simulink model "simulink_mppt_model"  (R2022b)
settings: Solver=VariableStepAuto  StartTime=0.0  StopTime=60  RelTol=1e-3  AbsTol=1e-3
model workspace (MAT data in the model file):
  Fsw = 40000
  Kc = 832.120994276
  batteryVoltage = 130
  deadTime = 5e-08
  wp = 45312.8685633
  wz = 3484.96300111
  zeroConductanceDef = 0.1
  zeroCurrentDef = 0.05
  zeroVoltageDef = 0.1
undefined symbols (not defined in the file): Ion, Lithium, sigbuilder_block
libraries: spsSeriesRLCBranchLib x5, dspstat3 x3, spsBatteryLib x1, spsControlledCurrentSourceLib x1, spsPVArrayLib x1, spsBoostConverterLib x1, spspowerguiLib x1
settings Model: ParameterArgumentNames=Fsw,deadTime,zeroCurrentDef  Creator=maxim  LastModifiedBy=maxim
settings SolverCC: AutoScaleAbsTol=off  AlgebraicLoopSolver=TrustRegion  MaxZcPerStep=1
settings DebuggingCC: UnconnectedInputMsg=warning  UnconnectedOutputMsg=warning  UnconnectedLineMsg=warning  SymbolicDimsDataTypeCodeGenerationDiagnostic=none  SFMachineParentedDataDiag=warning
settings ModelReferenceCC: EnableRefExpFcnMdlSchedulingChecks=on
settings SFSimCC: CustomCodeUndefinedFunction=UseInterfaceOnly  SimTargetLang=C++
settings RTWCC: DLArmComputeVersion=19.05
settings SimscapeCC: SimscapeLogType=all  SimscapeLogSimulationStatistics=on  SimscapeLogDataHistory=10000

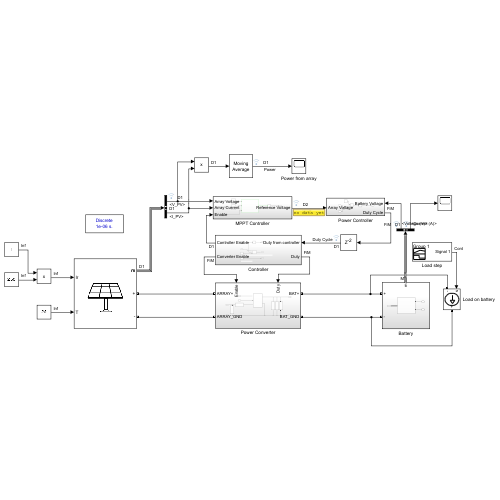
[thumbnail: Simulink's stored preview of the top-level diagram]
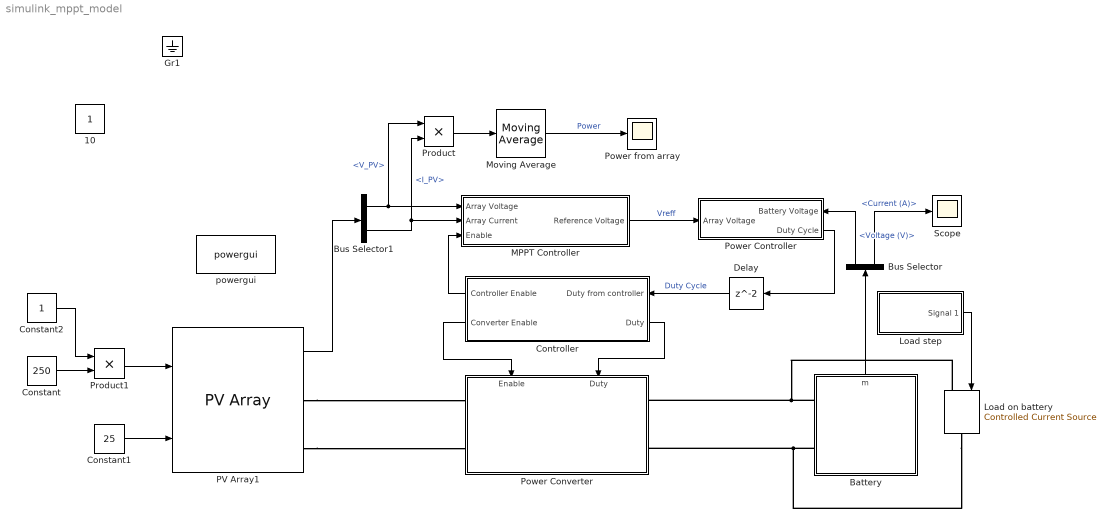
== system simulink_mppt_model ==
  Battery : Subsystem
      settings: PortSchema="{\"entries\":[{\"content\":{\"sides\":[{\"content\":{\"connectorIds\":[]},\"type\":\"ConnectorPlacement.EquallySpacedRectSide\",\"uuid\":\"681b39d9-76c9-4b82-8fbc-7b82f9fdea89\"},{\"content\":{\"connectorIds\":[\"RConn1\",\"RConn2\"],\"side\":\"RIGHT\"},\"type\":\"ConnectorPlacement.EquallySpacedRectSide\",\"uuid\":\"fad72295-eee8-4844-9071-ef3ebf9b61ad\"},{\"content\":{\"connectorIds\":[\"Out1\"],\"side\":\"TOP\"},\"type\":\"ConnectorPlacement.EquallySpacedRectSide\",\"uuid\":\"96a3c77e-3e0f-4d74-bbf8-3e2f46c7b130\"}]},\"type\":\"ConnectorPlacement.EquallySpacedConnector\",\"uuid\":\"ba8c3275-7e6c-45ac-aedb-539305cfe3f9\"}],\"packageUris\":[\"http://schema.mathworks.com/mf0/Connector/R2020b\"],\"version\":\"1.0\"}"
  Bus Selector : BusSelector  OutputSignals=Voltage (V),Current (A)
  Bus Selector1 : BusSelector  OutputSignals=V_PV,I_PV
  Constant : Constant  Value=250
  Constant1 : Constant  Value=25
  Constant2 : Constant
  Controller : Subsystem
      settings: PortSchema="{\"entries\":[{\"content\":{\"sides\":[{\"content\":{\"connectorIds\":[\"Out2\",\"Out3\"]},\"type\":\"ConnectorPlacement.EquallySpacedRectSide\",\"uuid\":\"2bf71abb-c260-460f-90aa-ee90c2514789\"},{\"content\":{\"connectorIds\":[\"In1\",\"Out1\"],\"side\":\"RIGHT\"},\"type\":\"ConnectorPlacement.EquallySpacedRectSide\",\"uuid\":\"98aef3cf-1e3e-4c29-bcc3-1b93ad6f6d73\"},{\"content\":{\"connectorIds\":[],\"side\":\"TOP\"},\"type\":\"ConnectorPlacement.EquallySpacedRectSide\",\"uuid\":\"494fa92e-9f19-4024-8cd4-71531be3e34f\"}]},\"type\":\"ConnectorPlacement.EquallySpacedConnector\",\"uuid\":\"d111867a-b07e-48e2-b097-48015141b267\"}],\"packageUris\":[\"http://schema.mathworks.com/mf0/Connector/R2020b\"],\"version\":\"1.0\"}"
  Delay : Delay
  Load on battery : spsControlledCurrentSourceLib/Controlled Current Source  Initialize=on  Source_Type=DC  Amplitude=0  Phase=0  Frequency=0  Measurements=Current
  Load step : Subsystem  Tag=STV Subsys  LoadFcn=sigbuilder_block('load');  StartFcn=sigbuilder_block('start');  StopFcn=sigbuilder_block('stop');  ClipboardFcn=sigbuilder_block('clipboard');  mask(Sigbuilder block){tuvar=[0:10]}
      mask help: Simulink:masks:SigbuilderBlock_MD
      mask init:
      | if ~strcmp(get_param(bdroot(gcbh),'SimulationStatus'),'stopped') tuvar = sigbuilder_block('maskInit'); end
      settings: CopyFcn=sigbuilder_block('copy');  DeleteFcn=sigbuilder_block('delete');  ModelCloseFcn=sigbuilder_block('modelClose');  PreSaveFcn=sigbuilder_block('preSave');  PauseFcn=sigbuilder_block('pause');  ContinueFcn=sigbuilder_block('continue');  NameChangeFcn=sigbuilder_block('namechange');  OpenFcn=sigbuilder_block('open',[440.25 198 550.5 399.75 ]);  CloseFcn=sigbuilder_block('close');
      mask Display: plot(0, 0, 100, 100,[2, 2, 32, 32, 2], [68, 8, 8, 68, 68],[32, 2], [38, 38], [32, 19, 2],[53, 60, 44], [32, 17, 17, 2],[16, 16, 31, 31]);txt = getActiveGroup(gcbh);text(2, 100, txt,'verticalAlignment', 'top');
  MPPT Controller : Subsystem
  Moving Average : dspstat3/Moving Average  Method=Sliding window  ForgettingFactorPort=off  SpecifyWindowLength=on  WindowLength=10  OverlapLength=9  AllowArbitraryInputLength=off  ForgettingFactor=0.9  SimulateUsing=Code generation
  PV Array1 : spsPVArrayLib/PV Array  Npar=1  Nser=100  PlotType=array @ 25 deg.C & specified irradiances  S_vec=[ 1000 500 400 300 200 100 50]  Temp_C_vec="[ 45 25  ]"  ModuleName=User-defined  PlotWhenSelected=off  Pm=3.3571  Ncell=1  Voc=0.71  Isc=6.08  Vm=0.59  Im=5.69  beta_Voc_pc=-0.36099  alpha_Isc_pc=0.102  beta_Voc=-0.002563  alpha_Isc=0.0062016  IL=6.0859  I0=2.2404e-10  nI=1.1511  Rsh=6.2378  Rs=0.0054799  RobustModel=off  RobustCellTemperature=313.3991  BAL=on  Tc=1e-6  Tfilter=5e-5
  Power Controller : Subsystem
      settings: PortSchema="{\"entries\":[{\"content\":{\"sides\":[{\"content\":{\"connectorIds\":[\"In1\"]},\"type\":\"ConnectorPlacement.EquallySpacedRectSide\",\"uuid\":\"eba48d98-7e83-4e3f-b762-8418122e8e33\"},{\"content\":{\"connectorIds\":[\"In2\",\"Out1\"],\"side\":\"RIGHT\"},\"type\":\"ConnectorPlacement.EquallySpacedRectSide\",\"uuid\":\"8bf8a633-4d87-4eab-b4cf-0c4a6a83ffe8\"},{\"content\":{\"connectorIds\":[],\"side\":\"TOP\"},\"type\":\"ConnectorPlacement.EquallySpacedRectSide\",\"uuid\":\"26ca6953-741f-43e9-aecb-d2f024797b97\"}]},\"type\":\"ConnectorPlacement.EquallySpacedConnector\",\"uuid\":\"d16115ba-55be-447b-aff6-c2745bc67311\"}],\"packageUris\":[\"http://schema.mathworks.com/mf0/Connector/R2020b\"],\"version\":\"1.0\"}"
  Power Converter : Subsystem
      settings: PortSchema="{\"entries\":[{\"content\":{\"sides\":[{\"content\":{\"connectorIds\":[\"LConn1\",\"LConn2\"]},\"type\":\"ConnectorPlacement.EquallySpacedRectSide\",\"uuid\":\"952598fd-f1ec-4ba0-8b7a-c65c9797eeff\"},{\"content\":{\"connectorIds\":[\"RConn1\",\"RConn2\"],\"side\":\"RIGHT\"},\"type\":\"ConnectorPlacement.EquallySpacedRectSide\",\"uuid\":\"a7adfdeb-ad62-4395-a0f0-2cb15f2f10ca\"},{\"content\":{\"connectorIds\":[\"In1\",\"In2\"],\"side\":\"TOP\"},\"type\":\"ConnectorPlacement.EquallySpacedRectSide\",\"uuid\":\"7d7424a5-d1fb-4a56-bd32-68ac8867628c\"},{\"content\":{\"connectorIds\":[],\"side\":\"BOTTOM\"},\"type\":\"ConnectorPlacement.EquallySpacedRectSide\",\"uuid\":\"0d675d46-7a1c-4391-83c9-5b80bbece1eb\"}]},\"type\":\"ConnectorPlacement.EquallySpacedConnector\",\"uuid\":\"24438d4f-f381-4eec-b9b7-2ef92542e692\"}],\"packageUris\":[\"http://schema.mathworks.com/mf0/Connector/R2020b\"],\"version\":\"1.0\"}"
  Power from array : Scope
  Product : Product
  Product1 : Product
  Scope : Scope
  powergui : spspowerguiLib/powergui  Priority=1  SimulationMode=Discrete  SampleTime=1e-6  frequency=60  Iterations=50  frequencyindice=0  Pbase=100e6  ErrMax=1e-4  UnitsV=kV  UnitsW=MW  buscounter=0  FunctionMessages=off  echomessages=off  EnableUseOfTLC=off  CurrentSourceSwitches=off  DisableSnubberDevices=off  DisableRonSwitches=off  DisableVfSwitches=off  DisplayEquations=off  AutomaticDiscreteSolvers=off  SolverType=Tustin/Backward Euler (TBE)  Interpol=off  ExternalGateDelay=off  methode=off  Ts=100  x0status=blocks  SPID=on  SwTol=0  HookPort=off  NonlinearTolerance=1e-4  nMaxIteration=100  ContinueOnMaxIteration=off  RestoreLinks=warning  ResistiveCurrentMeasurement=off  Frange=[0:2:500]  Ylog=off  Xlog=on  ShowGrid=off  save=off  variable=ZData  structure=0  ZoomFFT=off  StartTime=0.0  cycles=1  DisplayStyle=1  fundamental=60  FreqAxis=off  MaxFrequency=1000  frequencyindicesteady=1  RmsSteady=1  display=off
  10 : Constant  IOType=siggen
  Gr1 : Ground  IOType=siggen
  wires:
  Constant1/1 -> PV Array1/2
  PV Array1/1 -> Bus Selector1/1
  Product1/1 -> PV Array1/1
  Constant/1 -> Product1/2
  Bus Selector/1 -> Power Controller/2(Battery Voltage)  "<Voltage (V)>"
  Power Controller/1(Duty Cycle) -> Delay/1
  Constant2/1 -> Product1/1
  Battery/1(m) -> Bus Selector/1
  Bus Selector1/2 -> Product/2, MPPT Controller/2(Array Current)  "<I_PV>"
  Bus Selector1/1 -> Product/1, MPPT Controller/1(Array Voltage)  "<V_PV>"
  Product/1 -> Moving Average/1
  Moving Average/1 -> Power from array/1  "Power"
  MPPT Controller/1(Reference Voltage) -> Power Controller/1(Array Voltage)  "Vreff"
  Delay/1 -> Controller/1(Duty from controller)  "Duty Cycle"
  Controller/2(Controller Enable) -> MPPT Controller/3(Enable)
  Controller/1(Duty) -> Power Converter/2(Duty)
  Controller/3(Converter Enable) -> Power Converter/1(Enable)
  Load step/1(Signal 1) -> Load on battery/1
  Bus Selector/2 -> Scope/1  "<Current (A)>"
  connections:
  PV Array1/RConn1 -- Power Converter/LConn1
  Battery/RConn1 -- Load on battery/LConn1 -- Power Converter/RConn1
  Battery/RConn2 -- Load on battery/RConn1 -- Power Converter/RConn2
  PV Array1/RConn2 -- Power Converter/LConn2

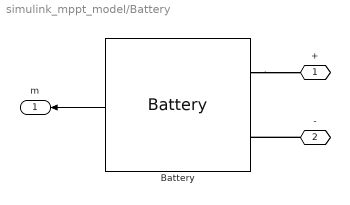
== system simulink_mppt_model/Battery ==
  Battery : spsBatteryLib/Battery  BatType=Lithium-Ion  ShowTempParam=off  ThermalPreset=no  ShowAgeParam=off  NomV=129.6  NomQ=155.25  SOC=60  Batt_Tr=0.01  PresetModel=on  MaxQ=155.25  MinV=97.2  FullV=150.8527  Dis_rate=67.5  R=0.0083478  Normal_OP=140.4  expZone="[140.018        7.6275]"  current=[6.5 13 32.5]  Units=Time  Tci=20  NomT=20  T2=-30  MaxQ2=4.8  FullV2=7.1  Normal_OP2=5.655  expZone2="[6.58           1]"  Rca=0.6  ti=2000  Dp=0  Neq0=0  Tsim=1e6  Ta1=25  Qeol=5.4*0.9  Reol=0.013333*1.2  Char_age=[2.3478, 3]  Dis_age=[2.3478, 10]  N1=1500  N2=10500  N3=1000  N4=1400  Ta2=45  N5=950
  + : PMIOPort  Side=Right
  - : PMIOPort  Port=2  Side=Right
  m : Outport
  wires:
  Battery/1 -> m/1
  connections:
  Battery/LConn1 -- +/RConn1
  -/RConn1 -- Battery/LConn2

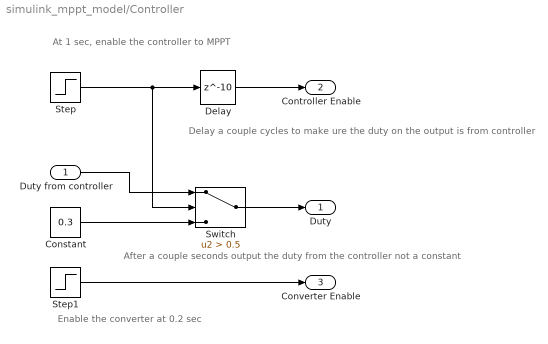
== system simulink_mppt_model/Controller ==
  note: At 1 sec, enable the controller to MPPT
  note: After a couple seconds output the duty from the controller not a constant
  note: Delay a couple cycles to make ure the duty on the output is from controller
  note: Enable the converter at 0.2 sec
  Duty from controller : Inport
  Constant : Constant  Value=0.3
  Delay : Delay  DelayLength=10
  Step : Step  SampleTime=0
  Step1 : Step  Time=0.2  Before=1  After=0  SampleTime=0
  Switch : Switch  Criteria=u2 > Threshold  Threshold=0.5  SaturateOnIntegerOverflow=off  InputSameDT=off
  Duty : Outport
  Controller Enable : Outport  Port=2
  Converter Enable : Outport  Port=3
  wires:
  Step/1 -> Switch/2, Delay/1
  Step1/1 -> Converter Enable/1
  Switch/1 -> Duty/1
  Constant/1 -> Switch/3
  Duty from controller/1 -> Switch/1
  Delay/1 -> Controller Enable/1

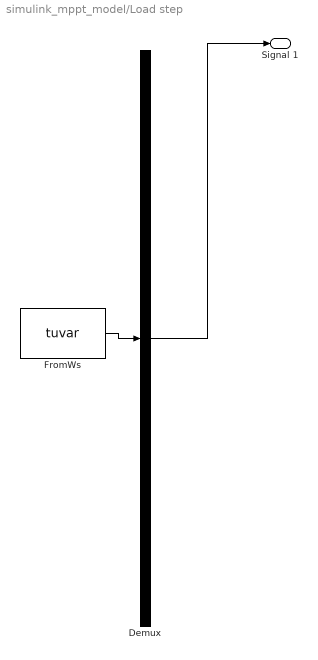
== system simulink_mppt_model/Load step ==
  Demux : Demux  Tag=STV Demux  Outputs=1
      settings: DisplayOption=none
  FromWs : FromWorkspace  Tag=STV FromWs  VariableName=tuvar
      SigBuilderData=|
      | common.afterFinalStr = 'Extrapolate'
      | common.sampleTime = 0
      | dataSet.timeRange = [0 10]
      | dataSet.name = 'Group 1'
      | sbobj.Groups.Name = 'Group 1'
      | sbobj.Groups.Signals.Name = 'Signal 1'
      | sbobj.Groups.Signals.XData = [0 2 2 3 3 10]
      | sbobj.Groups.Signals.YData = [0 0 30 30 7.4 7.6]
  Signal 1 : Outport  Tag=STV Outport
  wires:
  Demux/1 -> Signal 1/1
  FromWs/1 -> Demux/1

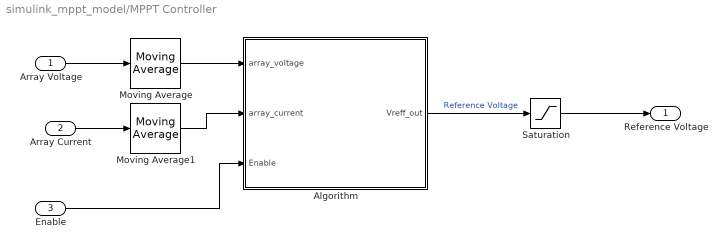
== system simulink_mppt_model/MPPT Controller ==
  Array Voltage : Inport
  Array Current : Inport  Port=2
  Enable : Inport  Port=3
  Algorithm : MATLAB Function  TreatAsAtomicUnit=on
  Moving Average : dspstat3/Moving Average  Method=Sliding window  ForgettingFactorPort=off  SpecifyWindowLength=on  WindowLength=10  OverlapLength=9  AllowArbitraryInputLength=off  ForgettingFactor=0.9  SimulateUsing=Code generation
  Moving Average1 : dspstat3/Moving Average  Method=Sliding window  ForgettingFactorPort=off  SpecifyWindowLength=on  WindowLength=10  OverlapLength=9  AllowArbitraryInputLength=off  ForgettingFactor=0.9  SimulateUsing=Code generation
  Saturation : Saturate  UpperLimit=100  LowerLimit=0
  Reference Voltage : Outport
  wires:
  Moving Average1/1 -> Algorithm/2(array_current)
  Array Voltage/1 -> Moving Average/1
  Algorithm/1(Vreff_out) -> Saturation/1  "Reference Voltage"
  Moving Average/1 -> Algorithm/1(array_voltage)
  Array Current/1 -> Moving Average1/1
  Saturation/1 -> Reference Voltage/1
  Enable/1 -> Algorithm/3(Enable)

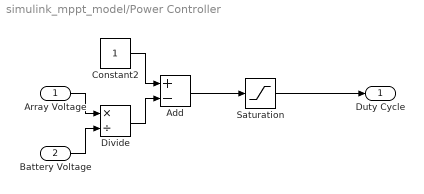
== system simulink_mppt_model/Power Controller ==
  Array Voltage : Inport
  Battery Voltage : Inport  Port=2
  Add : Sum  Inputs=+-
  Constant2 : Constant
  Divide : Product  Inputs=*/
  Saturation : Saturate  UpperLimit=0.9  LowerLimit=0
  Duty Cycle : Outport
  wires:
  Constant2/1 -> Add/1
  Battery Voltage/1 -> Divide/2
  Array Voltage/1 -> Divide/1
  Divide/1 -> Add/2
  Add/1 -> Saturation/1
  Saturation/1 -> Duty Cycle/1

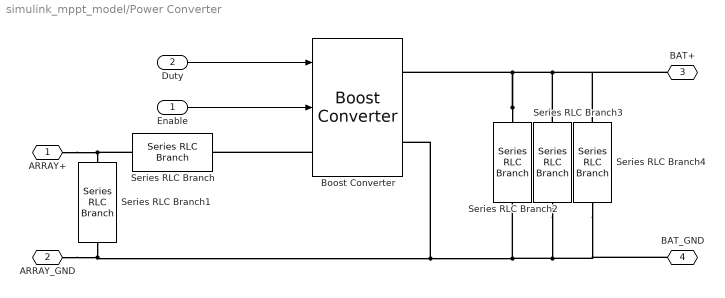
== system simulink_mppt_model/Power Converter ==
  Enable : Inport
  Duty : Inport  Port=2
  Boost Converter : spsBoostConverterLib/Boost Converter  ModelType=Average model (D-controlled)  Ron=1e-3  Rs=1e6  Cs=inf  Vforward=[0,0]  Ron_Diode=1e-3  Rs_Diode=1e6  Cs_Diode=inf  Vf_Diode=1e-3  Rs_CurrentSource=inf  Ron_ACsource=1e-3
      settings: LibrarySourceBlock=sps_lib/Power Electronics/Boost Converter
  Series RLC Branch : spsSeriesRLCBranchLib/Series RLC Branch  LConnTagsString=__new0  RConnTagsString=__new0  BranchType=RL  Resistance=0.064  Inductance=418e-6  SetiL0=on  InitialCurrent=2  Capacitance=1e-6  Setx0=off  InitialVoltage=0  Measurements=Branch current
  Series RLC Branch1 : spsSeriesRLCBranchLib/Series RLC Branch  LConnTagsString=__new0  RConnTagsString=__new0  BranchType=RC  Resistance=0.099  Inductance=1e-3  SetiL0=off  InitialCurrent=0  Capacitance=680*10^-6  Setx0=on  InitialVoltage=60  Measurements=None
  Series RLC Branch2 : spsSeriesRLCBranchLib/Series RLC Branch  LConnTagsString=__new0  RConnTagsString=__new0  BranchType=RC  Resistance=0.099  Inductance=1e-3  SetiL0=off  InitialCurrent=0  Capacitance=680*10^-6  Setx0=on  InitialVoltage=140  Measurements=Branch current
  Series RLC Branch3 : spsSeriesRLCBranchLib/Series RLC Branch  LConnTagsString=__new0  RConnTagsString=__new0  BranchType=RC  Resistance=0.099  Inductance=1e-3  SetiL0=off  InitialCurrent=0  Capacitance=680*10^-6  Setx0=on  InitialVoltage=140  Measurements=Branch current
  Series RLC Branch4 : spsSeriesRLCBranchLib/Series RLC Branch  LConnTagsString=__new0  RConnTagsString=__new0  BranchType=RC  Resistance=0.005  Inductance=1e-3  SetiL0=off  InitialCurrent=0  Capacitance=680*10^-9  Setx0=on  InitialVoltage=140  Measurements=Branch current
  ARRAY+ : PMIOPort  Side=Left
  ARRAY_GND : PMIOPort  Port=2  Side=Left
  BAT+ : PMIOPort  Port=3  Side=Right
  BAT_GND : PMIOPort  Port=4  Side=Right
  wires:
  Enable/1 -> Boost Converter/2
  Duty/1 -> Boost Converter/1
  connections:
  Series RLC Branch2/LConn1 -- Boost Converter/RConn1 -- Series RLC Branch4/LConn1 -- BAT+/RConn1 -- Series RLC Branch3/LConn1
  Boost Converter/LConn1 -- Series RLC Branch/RConn1
  Series RLC Branch/LConn1 -- ARRAY+/RConn1 -- Series RLC Branch1/LConn1
  ARRAY_GND/RConn1 -- BAT_GND/RConn1 -- Series RLC Branch4/RConn1 -- Series RLC Branch3/RConn1 -- Series RLC Branch2/RConn1 -- Boost Converter/RConn2 -- Series RLC Branch1/RConn1

== matlab function simulink_mppt_model/MPPT Controller/Algorithm ==
  settings: updateMethod=DISCRETE  sampleTime=1/200
  data: array_voltage input; array_current input; Vreff_out output; Enable input
function Vreff_out = mppt(array_voltage, array_current, Enable)


perterbAmount = 0.1;

persistent Vreff;
% persistent prevMaxPowerPointVoltage;
% persistent prevMaxPowerPointCurrent;
% 
% persistent zeroVoltageTolerance;
% persistent zeroCurrentTolerance;
% persistent zeroConductanceTolerance;

persistent prevVoltage;
persistent prevPower;
persistent direction;


if isempty(Vreff)
    Vreff = 20;
end

% 
% if isempty(prevMaxPowerPointCurrent)
%     prevMaxPowerPointCurrent = 0;
% end
% 
% if isempty(zeroVoltageTolerance)
%     zeroVoltageTolerance = 0.001;
% end
% 
% if isempty(zeroCurrentTolerance)
%     zeroCurrentTolerance = 0.02;
% end
% 
% if isempty(zeroConductanceTolerance)
%     zeroConductanceTolerance = 0.01;
% end

if isempty(prevPower)
    prevPower = 0;
end
if isempty(direction)
    direction = 1;
end
if isempty(prevVoltage)
    prevVoltage = 0;
end


% 
% deltaV = array_voltage - prevMaxPowerPointVoltage;
% deltaI = array_current - prevMaxPowerPointCurrent;

% if (abs(deltaV) < zeroVoltageTolerance)
%     if (abs(deltaI) < zeroCurrentTolerance)
%         duty = duty;
%     else
%         if (deltaI > 0)
%             duty = duty + 0.01; %algorithmOutput::decreaseInputVoltage
%         else
%             duty = duty - 0.01; %algorithmOutput::increaseInputVoltage
%         end
%     end
% else
%     if (abs(array_current / array_voltage + deltaI / deltaV) < zeroCurrentTolerance)
%         duty = duty;
%     else
%         if (array_current / array_voltage > -1 * (deltaI / deltaV))
%             duty = duty - 0.01; %algorithmOutput::increaseInputVoltage
%         else
%             duty = duty + 0.01; %algorithmOutput::decreaseInputVoltage
%         end
%     end
% end
% 
% prevMaxPowerPointVoltage = array_voltage;
% prevMaxPowerPointCurrent = array_current;

if(Enable ~= 1)
%%% Don't do anything if not enabled
end

curPower = array_voltage*array_current;

if(curPower > prevPower) 
    if (array_voltage > prevVoltage) 
        Vreff = Vreff + perterbAmount;
    else 
        Vreff = Vreff - perterbAmount;    
    end
else
    if (array_voltage > prevVoltage)
        Vreff = Vreff - perterbAmount;
    else 
        Vreff = Vreff + perterbAmount;    
    end
end

prevVoltage = array_voltage;
prevPower = curPower;

% if(array_voltage < 20 && array_voltage*array_current < 20)
%     duty = 0;
% else
%     duty = max(duty, 0);
% end

Vreff_out = Vreff;
